simulink model "fir_ssr"  (R2025a)
settings: Solver=VariableStepAuto  StartTime=0.0  StopTime=5000  RelTol=1e-3
PreLoadFcn:
  | xmcCheckSlxPath(bdroot)
  | SSR4_init
InitFcn:
  | xmcCheckSlxPath(bdroot)
  | SSR4_init;
values from neighbouring files (symbols this model uses):
  N = Ntaps - 1    [CreateFilter.m]    (also in SSR4_init.m = 2048; fir_ssr_init.m = 8192)
  S = sum(round(C0))    [NormalizeCoef.m]
  SHIFT_ACC = 15    [SSR4_init.m]    (also in fir_ssr_init.m)
  Taps = NormalizeCoef(UTaps,32768)    [SSR4_init.m]    (also in fir_ssr_init.m)
undefined symbols (not defined in the file or in its folder): None, vsva2197, xcvc1902
libraries: aieBasic x8, aieUtilities x4, dspobslib x1, aieDSP x1, simulink x1, vmcUtilities x1
settings Model: Creator=oliviert  LastModifiedBy=sdegala
settings SolverCC: AlgebraicLoopSolver=TrustRegion
settings DebuggingCC: UnconnectedInputMsg=warning  UnconnectedOutputMsg=warning  UnconnectedLineMsg=warning
settings ModelReferenceCC: EnableRefExpFcnMdlSchedulingChecks=on
settings RTWCC: GPUComputeCapability=3.5  DLArmComputeVersion=19.05

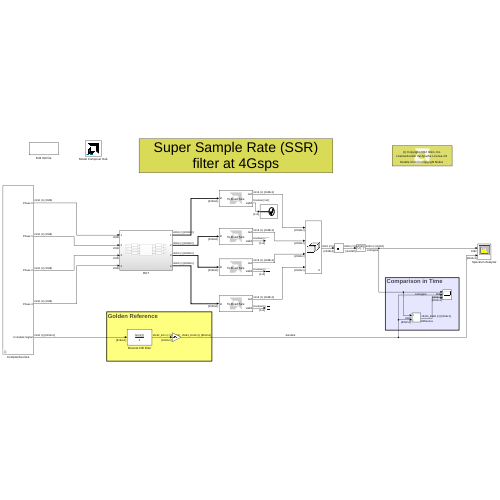
[thumbnail: Simulink's stored preview of the top-level diagram]
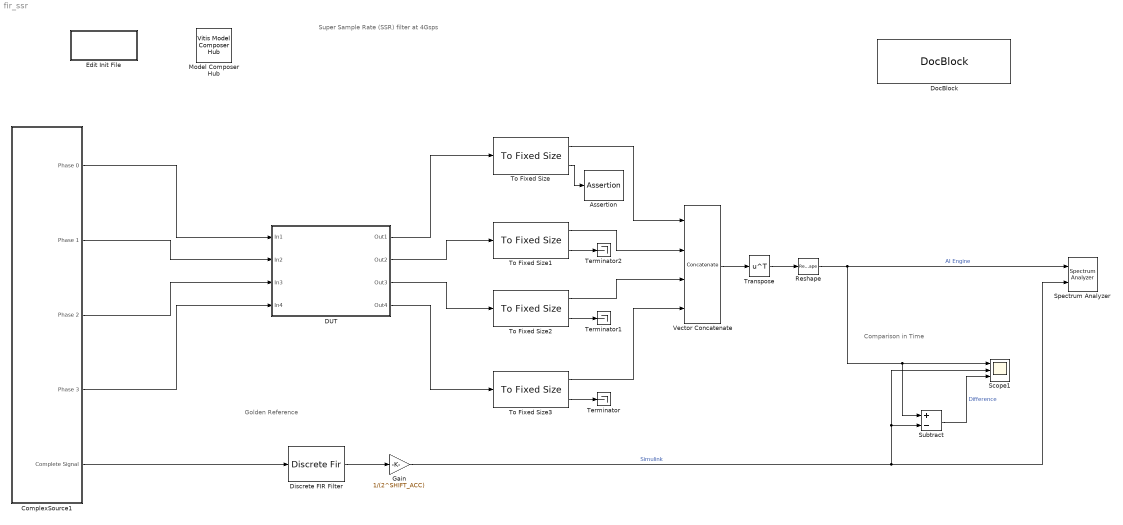
== system fir_ssr ==
  note: Comparison in Time
  note: Golden Reference
  note: Super Sample Rate (SSR) filter at 4Gsps
  Assertion : Assertion
  ComplexSource1 : Subsystem  mask{s=0}
      mask prompts: s "Seed"
  DUT : Subsystem
  Discrete FIR Filter : DiscreteFir  Coefficients=Taps  InputProcessing=Columns as channels (frame based)
  DocBlock : simulink/Model-Wide Utilities/DocBlock  DocumentType=Text  mask(DocBlock){}
      content=|
      | ///////////////////////////////////////////////////////////////////////////
      | // Copyright 2020 Xilinx
      | //
      | // Licensed under the Apache License, Version 2.0 (the "License");
      | // you may not use this file except in compliance with the License.
      | // You may obtain a copy of the License at
      | //
      | // http://www.apache.org/licenses/LICENSE-2.0
      | //
      | // Unless required by applicable law or agreed to in writing, software
      | // distributed under the License is distributed on an "AS IS" BASIS,
      | // WITHOUT WARRANTIES OR CONDITIONS OF ANY KIND, either express or implied.
      | // See the License for the specific language governing permissions and
      | // limitations under the License.
      | ///////////////////////////////////////////////////////////////////////////
      mask Display:
      | xmcDrawBlockIcon();
      | disp(['{\fontsize{10pt}(c) Copyright 2022' ' Xilinx, Inc.}\newline \newline '],'texmode','on');
      | disp('{\fontsize{10pt}Licensed under the Apache License 2.0}','texmode','on');
      | disp('\newline \newline \newline{\fontsize{10pt}Double Click for Copyright Notice}','texmode','on');
  Edit Init File : Subsystem
      settings: OpenFcn=edit('SSR4_init.m');
  Gain : Gain  Gain=1/(2^SHIFT_ACC)
  Model Composer Hub : vmcUtilities/Vitis Model Composer Hub  Tag=genX  CodeGeneration=off  SubsystemName=DUT  BlockHierPath=fir_ssr/DUT  SubsystemType=AIENode  AIEArrayConfig=Use entire AIE array  StartColumn=1  NumberOfColumns=1  TargetDirectory=./code  exportDesign=on  analyzeDesign=off  validateDesignOnHw=off  ExportType=AI Engines  IpVendor=xilinx.com  IpLibrary=hls  IpVersion=1.0  IpHWLanguage=Verilog  AieCompilerOptions={}  AieSimulatorOptions={}  CreateTestbench=on  TestbenchStackSize=10  RunRtlSim=off  RunCSim=off  RunAieSim=on  AieSimTimeout=50000  RunAieSimProfiling=off  LaunchVitisAnalyzer=off  PlotOutput=on  RunX86Sim=off  X86SimTimeout=10  GenHwImage=off  GenLibadfXo=off  GenHwValidationCode=off  PlatformType=Specify Platform  Platform=/proj/xbuilds/SWIP/9999.0_0818_1732/installs/lin64/2025.2/Vitis/base_platforms/xilinx_vck190_base_202520_1/xilinx_vck190_base_202520_1.xpfm  HwSystemType=Baremetal  HwValidationTarget=hw  ProjDevice=Versal VCK190 Evaluation Platform (xcvc1902-vsva2197-2MP-e-S)  ProjDevicePart=xcvc1902-vsva2197-2MP-e-S  AIEType=AIE  SamplePeriod=-1  ClockFrequency=200  DataPathParallelism=1  xilinxfamily=versalaicore  part=xcvc1902  speed=-2MP-e-S  package=vsva2197  directory=./netlist  testbench=off  incr_netlist=off  synthesis_tool=Vivado  clock_wrapper=Clock Enables  dbl_ovrd=According to Block Masks  dcm_input_clock_period=10  sysclk_period=10  simulink_period=1  eval_field=0  IPInfoJsonString="{\"DUTSubsystemName\":\"DUT\",\"AIESubsystem\":{\"SubsystemName\":\"DUT\",\"TargetDirectory\":\"./code\",\"AIEArrayConfig\":\"Use entire AIE array\",\"StartColumn\":\"0\",\"NumberOfColumns\":\"1\"},\"SubsystemTag\":\"AIENode\"}"  LogFileName=/proj/xhdhdstaff5/sdegala/Head1/HEAD/VMC_2025_2_July/Examples/AIENGINE/DSPlib/fir_ssr/code/model_composer.log  NThreads=4  IPConfigFile=/tmp/vmctmp-6835010160091439353/fir_ssr_ipconfig.json
  Reshape : Reshape
  Scope1 : Scope  NumInputPorts=3
      settings: ActiveDisplayYMinimum=-27332.375  ActiveDisplayYMaximum=27161.375  DataLoggingVariableName=ScopeData2
  Spectrum Analyzer : SpectrumAnalyzer  NumInputPorts=2  WindowPosition=[1494.000000,429.000000,422.000000,270.000000,]  Visible=on  ScopeFrameLocation=window  Method=Welch  SampleRate=8  Span=8  StartFrequency=-4  StopFrequency=4  AveragingMethod=Exponential  YLimits=[-16.1576 97.892]  ShowLegend=on  ChannelNames="[\"\"]"  AllowFFTLengthLessThanSamplesPerUpdate=on  DefaultConfigurationName=spbscopes.SpectrumAnalyzerBlockCfg
  Subtract : Sum  Inputs=+-
  Terminator : Terminator
  Terminator1 : Terminator
  Terminator2 : Terminator
  To Fixed Size{,1..3} (4 alike) : aieUtilities/To Fixed Size  Mode=Produce a valid output signal  OutputSize=Inherit: Same as input  CopyMethod=Buffer samples to form output  HasStatusOutput=off
  Transpose : Math  Operator=transpose
  Vector Concatenate : Concatenate  NumInputs=4  Mode=Multidimensional array  ConcatenateDimension=2
  wires:
  DUT/2(Out2) -> To Fixed Size1/1
  To Fixed Size1/1 -> Vector Concatenate/2
  Reshape/1 -> Spectrum Analyzer/1, Subtract/1, Scope1/1  "AI Engine"
  DUT/1(Out1) -> To Fixed Size/1
  Subtract/1 -> Scope1/3  "Difference"
  Vector Concatenate/1 -> Transpose/1
  To Fixed Size3/1 -> Vector Concatenate/4
  To Fixed Size2/1 -> Vector Concatenate/3
  Transpose/1 -> Reshape/1
  To Fixed Size/1 -> Vector Concatenate/1
  Discrete FIR Filter/1 -> Gain/1
  DUT/3(Out3) -> To Fixed Size2/1
  Gain/1 -> Spectrum Analyzer/2, Subtract/2, Scope1/2  "Simulink"
  DUT/4(Out4) -> To Fixed Size3/1
  ComplexSource1/3(Phase 2) -> DUT/3(In3)
  ComplexSource1/4(Phase 3) -> DUT/4(In4)
  ComplexSource1/1(Phase 0) -> DUT/1(In1)
  ComplexSource1/2(Phase 1) -> DUT/2(In2)
  ComplexSource1/5(Complete Signal) -> Discrete FIR Filter/1
  To Fixed Size/2 -> Assertion/1
  To Fixed Size3/2 -> Terminator/1
  To Fixed Size2/2 -> Terminator1/1
  To Fixed Size1/2 -> Terminator2/1

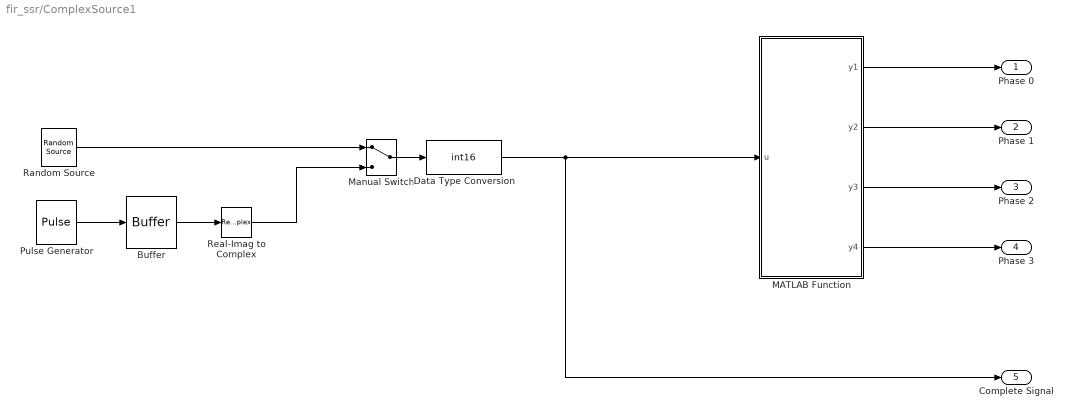
== system fir_ssr/ComplexSource1 ==
  Buffer : Buffer  N=N*4  OutputFrames=off
  Data Type Conversion : DataTypeConversion  OutDataTypeStr=int16  SaturateOnIntegerOverflow=off  RndMeth=Floor
  MATLAB Function : MATLAB Function  TreatAsAtomicUnit=on
  Manual Switch : ManualSwitch
  Pulse Generator : DiscretePulseGenerator  Amplitude=20000  Period=32 + 40*5  PhaseDelay=32  SampleTime=1/8
  Random Source : dspobslib/Random Source  SrcType=Uniform  NormMethod=Ziggurat  CltLength=12  MinVal=-20000  MaxVal=20000  MeanVal=0  VarVal=1  RepMode=Specify seed  rawSeed=s  IsInherit=off  SampMode=Discrete  SampTime=1/8  SampFrame=4*N  DataType=Double  OutComplex=Complex  OutputFrames=off
  Real-Imag to Complex : RealImagToComplex  Input=Real
  Phase 0 : Outport
  Phase 1 : Outport  Port=2
  Phase 2 : Outport  Port=3
  Phase 3 : Outport  Port=4
  Complete Signal : Outport  Port=5
  wires:
  MATLAB Function/1(y1) -> Phase 0/1
  MATLAB Function/2(y2) -> Phase 1/1
  MATLAB Function/3(y3) -> Phase 2/1
  MATLAB Function/4(y4) -> Phase 3/1
  Real-Imag to Complex/1 -> Manual Switch/2
  Pulse Generator/1 -> Buffer/1
  Data Type Conversion/1 -> Complete Signal/1, MATLAB Function/1(u)
  Buffer/1 -> Real-Imag to Complex/1
  Manual Switch/1 -> Data Type Conversion/1
  Random Source/1 -> Manual Switch/1

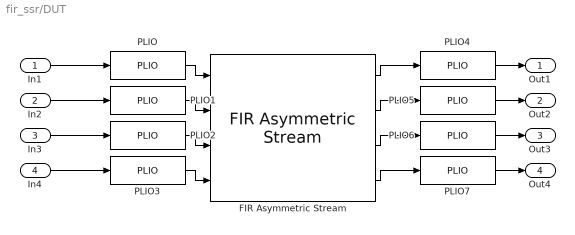
== system fir_ssr/DUT ==
  In1 : Inport
  In2 : Inport  Port=2
  In3 : Inport  Port=3
  In4 : Inport  Port=4
  FIR Asymmetric Stream : aieDSP/FIR Asymmetric Stream  data_type=cint16  coef_type=cint16  use_coeff_reload=off  dual_ip=off  num_outputs=off  coeff=Taps  fir_length=28  input_window_size=N*4  shift_val=SHIFT_ACC  rnd_mode=Round to positive infinity  sat_mode=0-None  ssr=NPHASES  casc_length=1  AIE_VARIANT=1  TP_API=1  blockJsonConstraints=[]  blockJsonConstraintsInternal=[]  spec=vmc_stream_fir_sr_asym.json  SerializedMaskParamNames=[]  SerializedMaskParamValues=[]  SerializedMaskParamVisibilities=[]  block_type=FIR Asymmetric Stream  SerializedMaskParamDataypes=typename|typename|uint|uint|uint|coef_type|uint|uint|uint|uint|uint|uint|uint|uint|uint  SerializedMaskParamEnumStrArr=0|0|0|0|0|0|0|0|0|Floor,Ceiling,Round to positive infinity,Round to negative infinity,Round symmetrical to infinity,Round symmetrical to zero,Round convergent to even,Round convergent to odd|0-None,1-Asymmetric,3-Symmetric|0|0|0|0  SerializedMaskParamEnumValArr=0|0|0|0|0|0|0|0|0|0,1,2,3,4,5,6,7|0,1,3|0|0|0|0  SerializedMaskParamVectorArr=0|0|0|0|0|1|0|0|0|0|0|0|0|0|0  SerializedMaskParamKeys=TT_DATA|TT_COEFF|TP_USE_COEFF_RELOAD|TP_DUAL_IP|TP_NUM_OUTPUTS|coeff|TP_FIR_LEN|TP_INPUT_WINDOW_VSIZE|TP_SHIFT|TP_RND|TP_SAT|TP_SSR|TP_CASC_LEN|AIE_VARIANT|TP_API
  PLIO{,1..7} (8 alike) : aieBasic/PLIO  PlioWidth=64  PlioFreqSpec=on  PlioFreq=PLIO_FREQ  ColLocation=0  channel=0  blockJsonConstraints=[]  deprecateConstraints=0
  Out1 : Outport
  Out2 : Outport  Port=2
  Out3 : Outport  Port=3
  Out4 : Outport  Port=4
  wires:
  In4/1 -> PLIO3/1
  In1/1 -> PLIO/1
  FIR Asymmetric Stream/4 -> PLIO7/1
  FIR Asymmetric Stream/1 -> PLIO4/1
  In2/1 -> PLIO1/1
  In3/1 -> PLIO2/1
  FIR Asymmetric Stream/2 -> PLIO5/1
  FIR Asymmetric Stream/3 -> PLIO6/1
  PLIO/1 -> FIR Asymmetric Stream/1
  PLIO1/1 -> FIR Asymmetric Stream/2
  PLIO2/1 -> FIR Asymmetric Stream/3
  PLIO3/1 -> FIR Asymmetric Stream/4
  PLIO4/1 -> Out1/1
  PLIO5/1 -> Out2/1
  PLIO6/1 -> Out3/1
  PLIO7/1 -> Out4/1

== system fir_ssr/Edit Init File ==

== matlab function fir_ssr/ComplexSource1/MATLAB Function ==
  data: u input; y1 output; y2 output; y3 output; y4 output
function [y1,y2,y3,y4] = fcn(u)

y1 = u(1:4:end);
y2 = u(2:4:end);
y3 = u(3:4:end);
y4 = u(4:4:end);
